simulink model "VehicleBody1DOFLongitudinalVDB"  (R2026b)
settings: Solver=VariableStepAuto
undefined symbols (not defined in the file): EnvAirTemp, EnvGrvty, PlntVehCGHgtAxl, PlntVehDstCGRearAxl, PlntVehHtchDst, PlntVehHtchHgtAxl, PlntVehHtchLatDst, PlntVehMass
libraries: autolibshared x1
settings Model: ModifiedByFormat=The MathWorks, Inc.  Creator=The MathWorks, Inc.  LastModifiedBy=The MathWorks, Inc.
settings OptimizationCC: ReuseModelBlockBuffer=off
settings DebuggingCC: SubsystemReferenceDiagnosticForUnitTest=warning

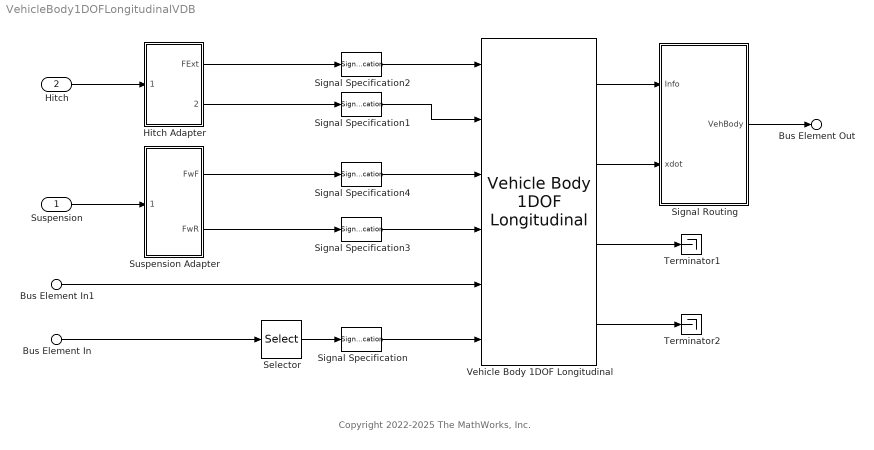
== system VehicleBody1DOFLongitudinalVDB ==
  note: Copyright 2022-2025 The MathWorks, Inc.
  Suspension : Inport
  Hitch : Inport  Port=2
  Bus Element In : Inport  Port=3  PortName=Env  Element=Wind
  Bus Element In1 : Inport  Port=3  PortName=Env  Element=Grade
  Hitch Adapter : Subsystem
  Selector : Selector  InputPortWidth=3  IndexOptions=Index vector (dialog)  Indices=[1]  OutputSizes=1
  Signal Routing : Subsystem
  Signal Specification : SignalSpecification  Unit=m/s
  Signal Specification1 : SignalSpecification  Unit=N*m
  Signal Specification2 : SignalSpecification  Unit=N
  Signal Specification3 : SignalSpecification  Unit=N
  Signal Specification4 : SignalSpecification  Unit=N
  Suspension Adapter : Subsystem
  Terminator1 : Terminator
  Terminator2 : Terminator
  Vehicle Body 1DOF Longitudinal : autolibshared/Vehicle Body 1DOF Longitudinal  VariantControl=SL  extFMode=on  extMMode=on  extTamb=off  wind3D=off  aMode=2  NF=PlntVehNumWhlFrntAxl  NR=PlntVehNumWhlRearAxl  m=PlntVehMass  a=PlntVehDstCGFrntAxl  b=PlntVehDstCGRearAxl  h=PlntVehCGHgtAxl  Cd=PlntVehAeroDragCff  Cl=PlntVehAeroLiftCff  Cpm=PlntVehAeroPitchCff  Af=PlntVehAeroFrntArea  x_o=PlntVehInitLongPos  xdot_o=PlntVehInitLongVel  Pabs=EnvAbsPrs  T=EnvAirTemp  g=EnvGrvty
      settings: LibrarySourceBlock=vehdynlibeom/Vehicle Body 1DOF Longitudinal
  Bus Element Out : Outport  PortName=VehBody
  wires:
  Bus Element In/1 -> Selector/1
  Selector/1 -> Signal Specification/1
  Suspension/1 -> Suspension Adapter/1(Suspension)
  Suspension Adapter/1(FwF) -> Signal Specification4/1
  Suspension Adapter/2(FwR) -> Signal Specification3/1
  Hitch Adapter/2(MExt) -> Signal Specification1/1
  Hitch/1 -> Hitch Adapter/1(Hitch)
  Hitch Adapter/1(FExt) -> Signal Specification2/1
  Signal Routing/1(VehBody) -> Bus Element Out/1
  Signal Specification2/1 -> Vehicle Body 1DOF Longitudinal/1
  Signal Specification1/1 -> Vehicle Body 1DOF Longitudinal/2
  Signal Specification4/1 -> Vehicle Body 1DOF Longitudinal/3
  Signal Specification3/1 -> Vehicle Body 1DOF Longitudinal/4
  Bus Element In1/1 -> Vehicle Body 1DOF Longitudinal/5
  Signal Specification/1 -> Vehicle Body 1DOF Longitudinal/6
  Vehicle Body 1DOF Longitudinal/1 -> Signal Routing/1(Info)
  Vehicle Body 1DOF Longitudinal/2 -> Signal Routing/2(xdot)
  Vehicle Body 1DOF Longitudinal/3 -> Terminator1/1
  Vehicle Body 1DOF Longitudinal/4 -> Terminator2/1

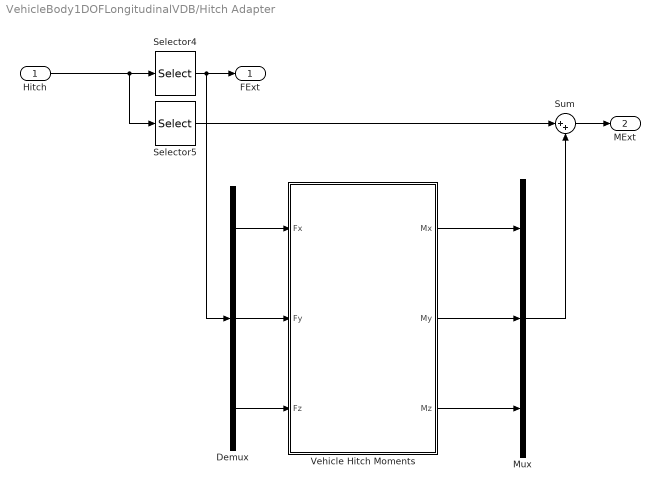
== system VehicleBody1DOFLongitudinalVDB/Hitch Adapter ==
  Hitch : Inport
  Demux : Demux  Outputs=3
  Mux : Mux  Inputs=3
  Selector4 : Selector  InputPortWidth=6  IndexOptions=Index vector (dialog)  Indices=[1:3]  OutputSizes=1
  Selector5 : Selector  InputPortWidth=6  IndexOptions=Index vector (dialog)  Indices=[4:6]  OutputSizes=1
  Sum : Sum  Inputs=|++
  Vehicle Hitch Moments : Subsystem  mask{h=PlntVehCGHgtAxl, dh=PlntVehHtchDst, hh=PlntVehHtchHgtAxl, hl=PlntVehHtchLatDst}
      mask prompts: h "vdynblks:vehdynTractorBody6Dof:blkPrm_h"; dh "vdynblks:vehdynTractorBody6Dof:blkPrm_dh"; hh "vdynblks:vehdynTractorBody6Dof:blkPrm_hh"; hl "vdynblks:vehdynTractorBody6Dof:blkPrm_hl"
      mask DialogControl h Prompt: Vertical distance from center of mass to axle plane, h [m]:
      mask DialogControl dh Prompt: Longitudinal distance from center of mass to hitch, dh [m]:
      mask DialogControl hh Prompt: Vertical distance from hitch to axle plane, hh [m]:
      mask DialogControl hl Prompt: Lateral distance from geometric centerline to hitch, hl [m]:
  FExt : Outport
  MExt : Outport  Port=2
  wires:
  Selector5/1 -> Sum/1
  Hitch/1 -> Selector5/1, Selector4/1
  Selector4/1 -> FExt/1, Demux/1
  Demux/1 -> Vehicle Hitch Moments/1(Fx)
  Demux/2 -> Vehicle Hitch Moments/2(Fy)
  Demux/3 -> Vehicle Hitch Moments/3(Fz)
  Vehicle Hitch Moments/1(Mx) -> Mux/1
  Vehicle Hitch Moments/2(My) -> Mux/2
  Vehicle Hitch Moments/3(Mz) -> Mux/3
  Sum/1 -> MExt/1
  Mux/1 -> Sum/2

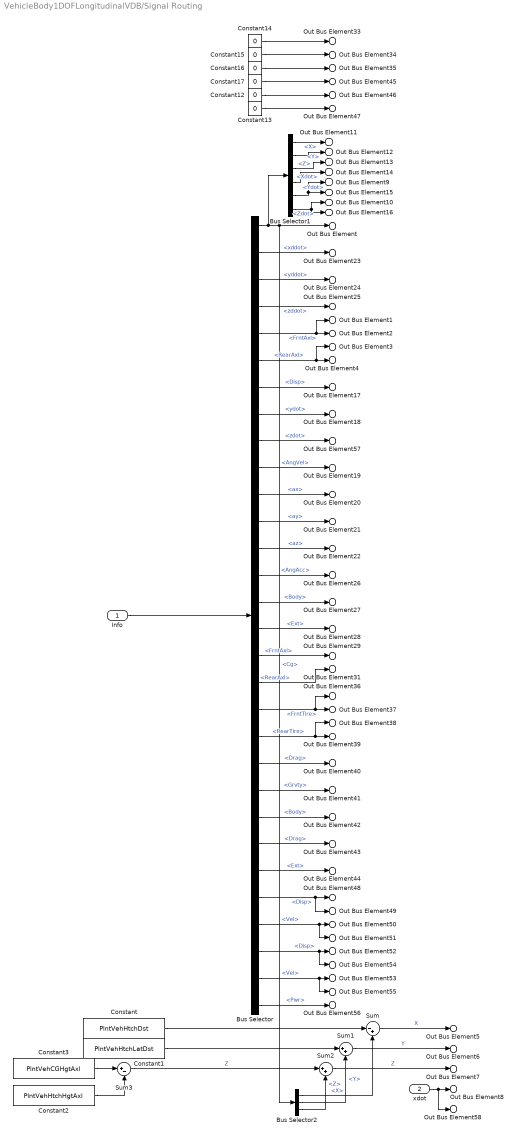
== system VehicleBody1DOFLongitudinalVDB/Signal Routing ==
  Info : Inport
  xdot : Inport  Port=2
  Bus Selector : BusSelector  OutputSignals=InertFrm.Cg,BdyFrm.Cg.Acc.xddot,BdyFrm.Cg.Acc.yddot,BdyFrm.Cg.Acc.zddot,InertFrm.FrntAxl,InertFrm.RearAxl,BdyFrm.Cg.Disp,BdyFrm.Cg.Vel.ydot,BdyFrm.Cg.Vel.zdot,BdyFrm.Cg.AngVel,BdyFrm.Cg.Acc.ax,BdyFrm.Cg.Acc.ay,BdyFrm.Cg.Acc.az,BdyFrm.Cg.AngAcc,BdyFrm.Forces.Body,BdyFrm.Forces.Ext,BdyFrm.Forces.FrntAxl,BdyFrm.Forces.RearAxl,BdyFrm.Forces.Tires.FrntTire,BdyFrm.Forces.Tires.RearTire,BdyFrm.Forces.Drag,BdyFrm.Forces.Grvty,BdyFrm.Moments.Body,BdyFrm.Moments.Drag,BdyFrm.Moments.Ext,BdyFrm.FrntAxl.Disp,BdyFrm.FrntAxl.Vel,BdyFrm.RearAxl.Disp,BdyFrm.RearAxl.Vel,BdyFrm.Pwr
  Bus Selector1 : BusSelector  OutputSignals=Disp.X,Disp.Y,Disp.Z,Vel.Xdot,Vel.Ydot,Vel.Zdot
  Bus Selector2 : BusSelector  OutputSignals=Disp.X,Disp.Y,Disp.Z
  Constant : Constant  Value=PlntVehHtchDst  SampleTime=-1
  Constant1 : Constant  Value=PlntVehHtchLatDst  SampleTime=-1
  Constant{12..17} (6 alike) : Constant  Value=0  SampleTime=-1
  Constant2 : Constant  Value=PlntVehHtchHgtAxl  SampleTime=-1
  Constant3 : Constant  Value=PlntVehCGHgtAxl  SampleTime=-1
  Sum : Sum  Inputs=|-+
  Sum1 : Sum  Inputs=|++
  Sum2 : Sum  Inputs=|++
  Sum3 : Sum  Inputs=|+-
  Out Bus Element : Outport  PortName=VehBody  Element=InertFrm.Cg
  Out Bus Element1 : Outport  PortName=VehBody  Element=InertFrm.FrntAxl.Lft
  Out Bus Element2 : Outport  PortName=VehBody  Element=InertFrm.FrntAxl.Rght
  Out Bus Element3 : Outport  PortName=VehBody  Element=InertFrm.RearAxl.Lft
  Out Bus Element4 : Outport  PortName=VehBody  Element=InertFrm.RearAxl.Rght
  Out Bus Element5 : Outport  PortName=VehBody  Element=InertFrm.Hitch.Disp.X
  Out Bus Element6 : Outport  PortName=VehBody  Element=InertFrm.Hitch.Disp.Y
  Out Bus Element7 : Outport  PortName=VehBody  Element=InertFrm.Hitch.Disp.Z
  Out Bus Element8 : Outport  PortName=VehBody  Element=InertFrm.Hitch.Vel.Xdot
  Out Bus Element9 : Outport  PortName=VehBody  Element=InertFrm.Hitch.Vel.Ydot
  Out Bus Element10 : Outport  PortName=VehBody  Element=InertFrm.Hitch.Vel.Zdot
  Out Bus Element11 : Outport  PortName=VehBody  Element=InertFrm.Geom.Disp.X
  Out Bus Element12 : Outport  PortName=VehBody  Element=InertFrm.Geom.Disp.Y
  Out Bus Element13 : Outport  PortName=VehBody  Element=InertFrm.Geom.Disp.Z
  Out Bus Element14 : Outport  PortName=VehBody  Element=InertFrm.Geom.Vel.Xdot
  Out Bus Element15 : Outport  PortName=VehBody  Element=InertFrm.Geom.Vel.Ydot
  Out Bus Element16 : Outport  PortName=VehBody  Element=InertFrm.Geom.Vel.Zdot
  Out Bus Element17 : Outport  PortName=VehBody  Element=BdyFrm.Cg.Disp
  Out Bus Element58 : Outport  PortName=VehBody  Element=BdyFrm.Cg.Vel.xdot
  Out Bus Element18 : Outport  PortName=VehBody  Element=BdyFrm.Cg.Vel.ydot
  Out Bus Element57 : Outport  PortName=VehBody  Element=BdyFrm.Cg.Vel.zdot
  Out Bus Element19 : Outport  PortName=VehBody  Element=BdyFrm.Cg.AngVel
  Out Bus Element20 : Outport  PortName=VehBody  Element=BdyFrm.Cg.Acc.ax
  Out Bus Element21 : Outport  PortName=VehBody  Element=BdyFrm.Cg.Acc.ay
  Out Bus Element22 : Outport  PortName=VehBody  Element=BdyFrm.Cg.Acc.az
  Out Bus Element23 : Outport  PortName=VehBody  Element=BdyFrm.Cg.Acc.xddot
  Out Bus Element24 : Outport  PortName=VehBody  Element=BdyFrm.Cg.Acc.yddot
  Out Bus Element25 : Outport  PortName=VehBody  Element=BdyFrm.Cg.Acc.zddot
  Out Bus Element26 : Outport  PortName=VehBody  Element=BdyFrm.Cg.AngAcc
  Out Bus Element27 : Outport  PortName=VehBody  Element=BdyFrm.Forces.Body
  Out Bus Element28 : Outport  PortName=VehBody  Element=BdyFrm.Forces.Ext
  Out Bus Element29 : Outport  PortName=VehBody  Element=BdyFrm.Forces.FrntAxl
  Out Bus Element31 : Outport  PortName=VehBody  Element=BdyFrm.Forces.RearAxl
  Out Bus Element33 : Outport  PortName=VehBody  Element=BdyFrm.Forces.Hitch.Fx
  Out Bus Element34 : Outport  PortName=VehBody  Element=BdyFrm.Forces.Hitch.Fy
  Out Bus Element35 : Outport  PortName=VehBody  Element=BdyFrm.Forces.Hitch.Fz
  Out Bus Element36 : Outport  PortName=VehBody  Element=BdyFrm.Forces.Tires.FrntTires.Lft
  Out Bus Element37 : Outport  PortName=VehBody  Element=BdyFrm.Forces.Tires.FrntTires.Rght
  Out Bus Element38 : Outport  PortName=VehBody  Element=BdyFrm.Forces.Tires.RearTires.Lft
  Out Bus Element39 : Outport  PortName=VehBody  Element=BdyFrm.Forces.Tires.RearTires.Rght
  Out Bus Element40 : Outport  PortName=VehBody  Element=BdyFrm.Forces.Drag
  Out Bus Element41 : Outport  PortName=VehBody  Element=BdyFrm.Forces.Grvty
  Out Bus Element42 : Outport  PortName=VehBody  Element=BdyFrm.Moments.Body
  Out Bus Element43 : Outport  PortName=VehBody  Element=BdyFrm.Moments.Drag
  Out Bus Element44 : Outport  PortName=VehBody  Element=BdyFrm.Moments.Ext
  Out Bus Element45 : Outport  PortName=VehBody  Element=BdyFrm.Moments.Hitch.Mx
  Out Bus Element46 : Outport  PortName=VehBody  Element=BdyFrm.Moments.Hitch.My
  Out Bus Element47 : Outport  PortName=VehBody  Element=BdyFrm.Moments.Hitch.Mz
  Out Bus Element48 : Outport  PortName=VehBody  Element=BdyFrm.FrntAxl.Lft.Disp
  Out Bus Element50 : Outport  PortName=VehBody  Element=BdyFrm.FrntAxl.Lft.Vel
  Out Bus Element49 : Outport  PortName=VehBody  Element=BdyFrm.FrntAxl.Rght.Disp
  Out Bus Element51 : Outport  PortName=VehBody  Element=BdyFrm.FrntAxl.Rght.Vel
  Out Bus Element52 : Outport  PortName=VehBody  Element=BdyFrm.RearAxl.Lft.Disp
  Out Bus Element53 : Outport  PortName=VehBody  Element=BdyFrm.RearAxl.Lft.Vel
  Out Bus Element54 : Outport  PortName=VehBody  Element=BdyFrm.RearAxl.Rght.Disp
  Out Bus Element55 : Outport  PortName=VehBody  Element=BdyFrm.RearAxl.Rght.Vel
  Out Bus Element56 : Outport  PortName=VehBody  Element=BdyFrm.Pwr
  wires:
  Bus Selector/9 -> Out Bus Element57/1  "<zdot>"
  Bus Selector/13 -> Out Bus Element22/1  "<az>"
  Bus Selector/12 -> Out Bus Element21/1  "<ay>"
  Constant13/1 -> Out Bus Element47/1
  Constant12/1 -> Out Bus Element46/1
  Constant17/1 -> Out Bus Element45/1
  Constant16/1 -> Out Bus Element35/1
  Constant15/1 -> Out Bus Element34/1
  Constant14/1 -> Out Bus Element33/1
  xdot/1 -> Out Bus Element8/1, Out Bus Element58/1
  Constant1/1 -> Sum1/1
  Sum1/1 -> Out Bus Element6/1  "Y"
  Sum/1 -> Out Bus Element5/1  "X"
  Constant2/1 -> Sum3/2
  Sum2/1 -> Out Bus Element7/1  "Z"
  Constant3/1 -> Sum3/1
  Sum3/1 -> Sum2/1  "Z"
  Constant/1 -> Sum/1
  Bus Selector2/2 -> Sum1/2  "<Y>"
  Bus Selector2/1 -> Sum/2  "<X>"
  Bus Selector2/3 -> Sum2/2  "<Z>"
  Info/1 -> Bus Selector/1
  Bus Selector/1 -> Out Bus Element/1, Bus Selector2/1, Bus Selector1/1  "<Cg>"
  Bus Selector/5 -> Out Bus Element1/1, Out Bus Element2/1  "<FrntAxl>"
  Bus Selector/6 -> Out Bus Element3/1, Out Bus Element4/1  "<RearAxl>"
  Bus Selector/15 -> Out Bus Element27/1  "<Body>"
  Bus Selector/16 -> Out Bus Element28/1  "<Ext>"
  Bus Selector/17 -> Out Bus Element29/1  "<FrntAxl>"
  Bus Selector/18 -> Out Bus Element31/1  "<RearAxl>"
  Bus Selector/19 -> Out Bus Element36/1, Out Bus Element37/1  "<FrntTire>"
  Bus Selector/20 -> Out Bus Element38/1, Out Bus Element39/1  "<RearTire>"
  Bus Selector/21 -> Out Bus Element40/1  "<Drag>"
  Bus Selector/22 -> Out Bus Element41/1  "<Grvty>"
  Bus Selector/23 -> Out Bus Element42/1  "<Body>"
  Bus Selector/24 -> Out Bus Element43/1  "<Drag>"
  Bus Selector/25 -> Out Bus Element44/1  "<Ext>"
  Bus Selector/30 -> Out Bus Element56/1  "<Pwr>"
  Bus Selector/26 -> Out Bus Element48/1, Out Bus Element49/1  "<Disp>"
  Bus Selector/27 -> Out Bus Element50/1, Out Bus Element51/1  "<Vel>"
  Bus Selector/28 -> Out Bus Element52/1, Out Bus Element54/1  "<Disp>"
  Bus Selector/29 -> Out Bus Element53/1, Out Bus Element55/1  "<Vel>"
  Bus Selector/7 -> Out Bus Element17/1  "<Disp>"
  Bus Selector/8 -> Out Bus Element18/1  "<ydot>"
  Bus Selector/11 -> Out Bus Element20/1  "<ax>"
  Bus Selector/14 -> Out Bus Element26/1  "<AngAcc>"
  Bus Selector/10 -> Out Bus Element19/1  "<AngVel>"
  Bus Selector/2 -> Out Bus Element23/1  "<xddot>"
  Bus Selector/3 -> Out Bus Element24/1  "<yddot>"
  Bus Selector/4 -> Out Bus Element25/1  "<zddot>"
  Bus Selector1/1 -> Out Bus Element11/1  "<X>"
  Bus Selector1/2 -> Out Bus Element12/1  "<Y>"
  Bus Selector1/3 -> Out Bus Element13/1  "<Z>"
  Bus Selector1/4 -> Out Bus Element14/1  "<Xdot>"
  Bus Selector1/5 -> Out Bus Element15/1, Out Bus Element9/1  "<Ydot>"
  Bus Selector1/6 -> Out Bus Element16/1, Out Bus Element10/1  "<Zdot>"

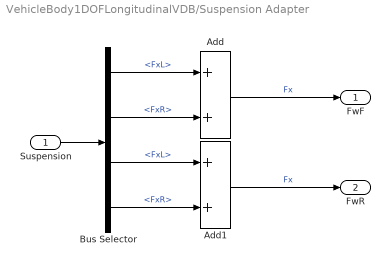
== system VehicleBody1DOFLongitudinalVDB/Suspension Adapter ==
  Suspension : Inport
  Add : Sum
  Add1 : Sum
  Bus Selector : BusSelector  OutputSignals=FrntSusp.FrntSuspWheel.Wheels.Fx.FxL,FrntSusp.FrntSuspWheel.Wheels.Fx.FxR,RearSusp.RearSuspWheel.Wheels.Fx.FxL,RearSusp.RearSuspWheel.Wheels.Fx.FxR
  FwF : Outport
  FwR : Outport  Port=2
  wires:
  Bus Selector/4 -> Add1/2  "<FxR>"
  Bus Selector/3 -> Add1/1  "<FxL>"
  Bus Selector/2 -> Add/2  "<FxR>"
  Bus Selector/1 -> Add/1  "<FxL>"
  Add/1 -> FwF/1  "Fx"
  Add1/1 -> FwR/1  "Fx"
  Suspension/1 -> Bus Selector/1

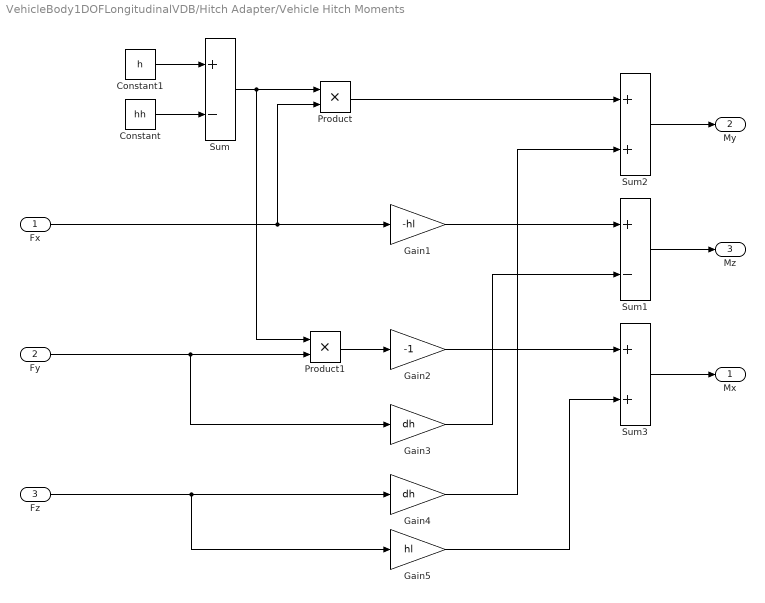
== system VehicleBody1DOFLongitudinalVDB/Hitch Adapter/Vehicle Hitch Moments ==
  Fx : Inport
  Fy : Inport  Port=2
  Fz : Inport  Port=3
  Constant : Constant  Value=hh  SampleTime=-1
  Constant1 : Constant  Value=h  SampleTime=-1
  Gain1 : Gain  Gain=-hl
  Gain2 : Gain  Gain=-1
  Gain3 : Gain  Gain=dh
  Gain4 : Gain  Gain=dh
  Gain5 : Gain  Gain=hl
  Product : Product
  Product1 : Product
  Sum : Sum  Inputs=+-
  Sum1 : Sum  Inputs=+-
  Sum2 : Sum
  Sum3 : Sum
  Mx : Outport
  My : Outport  Port=2
  Mz : Outport  Port=3
  wires:
  Fy/1 -> Gain3/1, Product1/2
  Product1/1 -> Gain2/1
  Sum/1 -> Product1/1, Product/1
  Product/1 -> Sum2/1
  Constant1/1 -> Sum/1
  Gain3/1 -> Sum1/2
  Fx/1 -> Product/2, Gain1/1
  Fz/1 -> Gain5/1, Gain4/1
  Sum2/1 -> My/1
  Constant/1 -> Sum/2
  Gain1/1 -> Sum1/1
  Gain4/1 -> Sum2/2
  Gain5/1 -> Sum3/2
  Gain2/1 -> Sum3/1
  Sum1/1 -> Mz/1
  Sum3/1 -> Mx/1
